simulink model "drive4ACC"  (R2018b)
settings: Solver=FixedStepAuto  StartTime=0.0  StopTime=inf  FixedStep=1/400  RelTol=1e-3  EnableMultiTasking=on
libraries: libcontrol x4, simulink x1
settings Model: ExtModeTrigDuration=100  Creator=Lenovo  LastModifiedBy=Lenovo
settings SolverCC: PositivePriorityOrder=on  AutoInsertRateTranBlk=on
settings OptimizationCC: EnhancedBackFolding=on  PassReuseOutputArgsAs=Individual arguments  MaxStackSize=64  OptimizeBlockOrder=speed  DifferentSizesBufferReuse=on  OptimizationCustomize=off
settings DebuggingCC: ParameterTunabilityLossMsg=error
settings HardwareCC: ProdBitPerPointer=32  ProdBitPerSizeT=32  ProdBitPerPtrDiffT=32  ProdLargestAtomicInteger=Long  ProdLargestAtomicFloat=Double  ProdWordSize=32  ProdHWDeviceType=ARM Compatible->ARM Cortex
settings SFSimCC: MATLABDynamicMemAlloc=off
settings RTWCC: SystemTargetFile=ert.tlc  HardwareBoard=BeagleBone Blue  TLCOptions="-aInlineSetEventsForThisBaseRateFcn=TLC_FALSE -aSuppressMultiTaskScheduler=TLC_FALSE  -aRateBasedStepFcn=0"  TemplateMakefile=ert_default_tmf  GenerateReport=on  Toolchain=GNU GCC BeagleBone Blue  IncludeHyperlinkInReport=on  LaunchReport=on  GenerateTraceInfo=on  GenerateTraceReport=on  GenerateTraceReportSl=on  GenerateTraceReportSf=on  GenerateTraceReportEml=on
settings CodeAppCC: ForceParamTrailComments=on  IgnoreCustomStorageClasses=off  OperatorAnnotations=on  SimulinkDataObjDesc=on  SFDataObjDesc=on  InsertBlockDesc=on
settings ERTTargetCC: SupportVariableSizeSignals=on

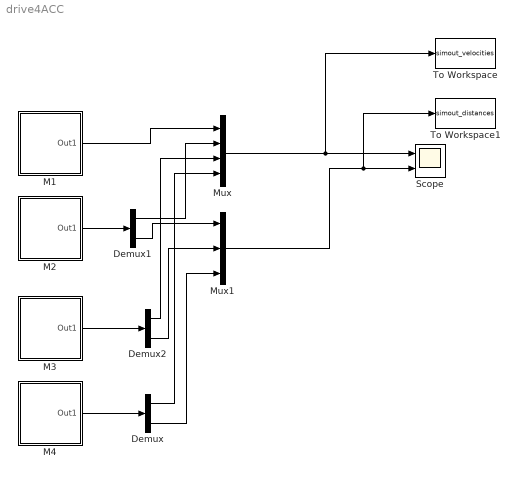
== system drive4ACC ==
  Demux : Demux  Outputs=2
  Demux1 : Demux  Outputs=2
  Demux2 : Demux  Outputs=2
  M1 : Subsystem
  M2 : Subsystem
  M3 : Subsystem
  M4 : Subsystem
  Mux : Mux
  Mux1 : Mux  Inputs=3
  Scope : Scope  NumInputPorts=2
  To Workspace : ToWorkspace  VariableName=simout_velocities  SaveFormat=Timeseries  SampleTime=-1
  To Workspace1 : ToWorkspace  VariableName=simout_distances  SaveFormat=Timeseries  SampleTime=-1
  wires:
  Mux/1 -> To Workspace/1, Scope/1
  Mux1/1 -> To Workspace1/1, Scope/2
  M1/1(Out1) -> Mux/1
  M2/1(Out1) -> Demux1/1
  M3/1(Out1) -> Demux2/1
  M4/1(Out1) -> Demux/1
  Demux2/2 -> Mux1/2
  Demux1/1 -> Mux/2
  Demux1/2 -> Mux1/1
  Demux2/1 -> Mux/3
  Demux/1 -> Mux/4
  Demux/2 -> Mux1/3

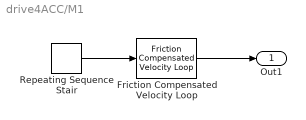
== system drive4ACC/M1 ==
  Friction Compensated Velocity Loop : libcontrol/Friction Compensated Velocity Loop  SystemSampleTime=-1
  Repeating Sequence Stair : simulink/Sources/Repeating Sequence Stair  OutValues=[0.8 0.3 0.8].'  tsamp=5  OutMin=[]  OutMax=[]  OutDataTypeStr=double  OutputDataTypeScalingMode=double  OutDataType=fixdt(0,8)  ConRadixGroup=Best Precision: Vector-wise  OutScaling=2^-12
  Out1 : Outport
  wires:
  Friction Compensated Velocity Loop/1 -> Out1/1
  Repeating Sequence Stair/1 -> Friction Compensated Velocity Loop/1

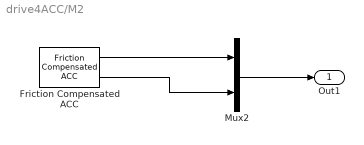
== system drive4ACC/M2 ==
  Friction Compensated ACC : libcontrol/Friction Compensated ACC  SystemSampleTime=-1
  Mux2 : Mux  Inputs=2
  Out1 : Outport
  wires:
  Friction Compensated ACC/1 -> Mux2/1
  Friction Compensated ACC/2 -> Mux2/2
  Mux2/1 -> Out1/1

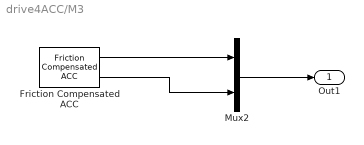
== system drive4ACC/M3 ==
  Friction Compensated ACC : libcontrol/Friction Compensated ACC  SystemSampleTime=-1
  Mux2 : Mux  Inputs=2
  Out1 : Outport
  wires:
  Friction Compensated ACC/1 -> Mux2/1
  Friction Compensated ACC/2 -> Mux2/2
  Mux2/1 -> Out1/1

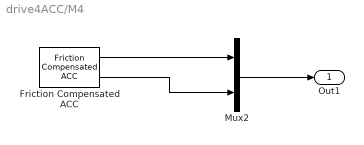
== system drive4ACC/M4 ==
  Friction Compensated ACC : libcontrol/Friction Compensated ACC  SystemSampleTime=-1
  Mux2 : Mux  Inputs=2
  Out1 : Outport
  wires:
  Friction Compensated ACC/1 -> Mux2/1
  Friction Compensated ACC/2 -> Mux2/2
  Mux2/1 -> Out1/1
